simulink library "lib_Convection_LamCoiledTube"  (R2015a)
settings: Solver=ode45  StartTime=0.0  StopTime=10.0  RelTol=1e-3
libraries: simulink x4
settings Model: Creator=jlkratz  LastModifiedBy=jlkratz

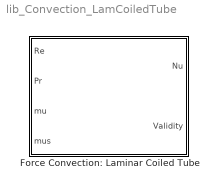
== system lib_Convection_LamCoiledTube ==
  Force Convection: Laminar Coiled Tube : Subsystem  mask(TSAT: Laminar Coiled Tube){DoC_M=0.1}
      mask prompts: DoC_M "DoC_M - Ratio of the diameter of the pipe flow cross-section to the diameter of the coils (D/C)"
      mask help:
      | This block estimates the average Nusselt number for a helically coiled tube with an internal flow. The correlation was provided by Shah and Joshi. Coiled tubes are sometimes used to enhance heat transfer without turbulence or additional surface area. It utilizes centrifugal forces within the flow which induces secondary flow that enhances heat transfer. The implemented correlation is valid for:
      |
      | 0.005 <= Pr <= 1600
      | 1 <= Re*(D/C)^(1/2) <= 1000
      |
      | The second contraint typically restricts use to laminar flow (Re < Re,c*(1 + 12*(D/C)^(1/2)), Re,c = ~2300). For turbulent flow the effects of secondary flow is minor and a straight pipe correlation for turbulent flow is more appropriate. Also, a straight pipe laminar flow correlation may suffice when C/D >= 20 in which case error is less than 10%. Note that the Reynolds number and ensuing heat transfer coefficient should be calculated using the diameter of the tube (D) as the characteristic length. See the block help menu for more details.
      mask Help: web(which('Convection_TSAT_LamCoiledTube.html'),'-helpbrowser')
      mask DialogControl Container3 Prompt: Parameters

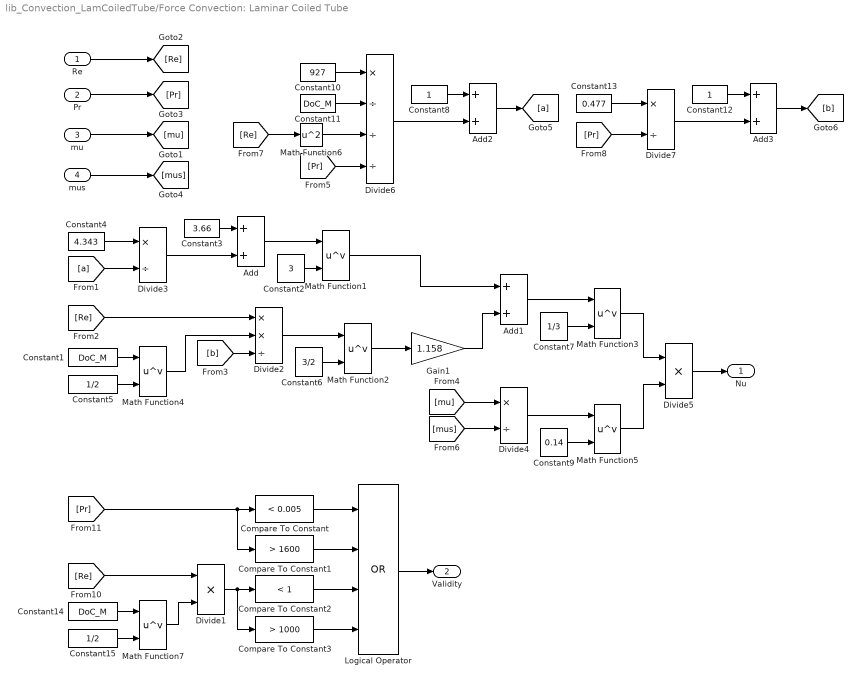
== system lib_Convection_LamCoiledTube/Force Convection: Laminar Coiled Tube ==
  Re : Inport
  Pr : Inport  Port=2
  mu : Inport  Port=3
  mus : Inport  Port=4
  Add{,1..3} (4 alike) : Sum
  Compare To Constant : simulink/Logic and Bit Operations/Compare To Constant  relop=<  const=0.005  OutDataTypeStr=boolean
  Compare To Constant1 : simulink/Logic and Bit Operations/Compare To Constant  relop=>  const=1600  OutDataTypeStr=boolean
  Compare To Constant2 : simulink/Logic and Bit Operations/Compare To Constant  relop=<  const=1  OutDataTypeStr=boolean
  Compare To Constant3 : simulink/Logic and Bit Operations/Compare To Constant  relop=>  const=1000  OutDataTypeStr=boolean
  Constant1 : Constant  Value=DoC_M
  Constant10 : Constant  Value=927
  Constant11 : Constant  Value=DoC_M
  Constant12 : Constant
  Constant13 : Constant  Value=0.477
  Constant14 : Constant  Value=DoC_M
  Constant15 : Constant  Value=1/2
  Constant2 : Constant  Value=3
  Constant3 : Constant  Value=3.66
  Constant4 : Constant  Value=4.343
  Constant5 : Constant  Value=1/2
  Constant6 : Constant  Value=3/2
  Constant7 : Constant  Value=1/3
  Constant8 : Constant
  Constant9 : Constant  Value=0.14
  Divide1 : Product  Inputs=**
  Divide2 : Product  Inputs=**/
  Divide3 : Product  Inputs=*/
  Divide4 : Product  Inputs=*/
  Divide5 : Product  Inputs=**
  Divide6 : Product  Inputs=*///
  Divide7 : Product  Inputs=*/
  Gain1 : Gain  Gain=1.158
  Logical Operator : Logic  Operator=OR  Inputs=4  AllPortsSameDT=off  OutDataTypeStr=boolean
  Math Function{1..5,7} (6 alike) : Math  Operator=pow  SaturateOnIntegerOverflow=on
  Math Function6 : Math  Operator=square  SaturateOnIntegerOverflow=on
  Nu : Outport
  Validity : Outport  Port=2
  wires:
  Logical Operator/1 -> Validity/1
  Compare To Constant3/1 -> Logical Operator/4
  Compare To Constant2/1 -> Logical Operator/3
  Compare To Constant1/1 -> Logical Operator/2
  Compare To Constant/1 -> Logical Operator/1
  [Pr] -> Compare To Constant/1, Compare To Constant1/1
  Divide1/1 -> Compare To Constant2/1, Compare To Constant3/1
  [Re] -> Divide1/1
  Math Function7/1 -> Divide1/2
  Constant15/1 -> Math Function7/2
  Constant14/1 -> Math Function7/1
  Add3/1 -> [b]
  Constant13/1 -> Divide7/1
  [Pr] -> Divide7/2
  Constant12/1 -> Add3/1
  Divide7/1 -> Add3/2
  Add2/1 -> [a]
  Constant8/1 -> Add2/1
  Divide6/1 -> Add2/2
  [Re] -> Math Function6/1
  Math Function6/1 -> Divide6/3
  Constant11/1 -> Divide6/2
  Constant10/1 -> Divide6/1
  Constant9/1 -> Math Function5/2
  Divide5/1 -> Nu/1
  Math Function5/1 -> Divide5/2
  Math Function3/1 -> Divide5/1
  Divide4/1 -> Math Function5/1
  [mus] -> Divide4/2
  [mu] -> Divide4/1
  mus/1 -> [mus]
  mu/1 -> [mu]
  Constant7/1 -> Math Function3/2
  Add1/1 -> Math Function3/1
  Gain1/1 -> Add1/2
  Math Function2/1 -> Gain1/1
  Constant6/1 -> Math Function2/2
  Divide2/1 -> Math Function2/1
  [b] -> Divide2/3
  Math Function4/1 -> Divide2/2
  [Re] -> Divide2/1
  Constant5/1 -> Math Function4/2
  Constant1/1 -> Math Function4/1
  Math Function1/1 -> Add1/1
  Add/1 -> Math Function1/1
  Divide3/1 -> Add/2
  [a] -> Divide3/2
  Constant4/1 -> Divide3/1
  [Pr] -> Divide6/4
  Constant3/1 -> Add/1
  Pr/1 -> [Pr]
  Re/1 -> [Re]
  Constant2/1 -> Math Function1/2
